simulink model "uasb_siso_simu"  (R2024b)
settings: Solver=VariableStepAuto  StartTime=0.0  StopTime=60  RelTol=1e-3
values from neighbouring files (symbols this model uses):
  A = blkdiag(A1, A2)    [generic_simo.m]    (also in uasb.m = [A1, zeros(3); uasb_identification.m = readmatrix('A2.csv'); uasb_siso.m = [-a_(2:end)', [1; 0]])
  B = [ ... (first row only)    [generic_simo.m]    (also in uasb.m = [B11(2:end), B12(2:end); uasb_identification.m = readmatrix('B2.csv'); uasb_siso.m = b')
  D = [D1 ... (first row only)    [generic_simo.m]    (also in uasb.m = [D1, zeros(3,1); uasb_siso.m = -a_(2:end)')
  delta = [1 -1]    [generic_simo.m]    (also in uasb.m = tf(1, delta, Ts, 'variable', 'z^-1'); uasb_siso.m = [1, -1])
  H = blkdiag(H1, H2)    [generic_simo.m]    (also in uasb.m = [H1, 0, 0, 0; uasb_siso.m = [1, 0])
  KE = K * E    [generic_simo.m]    (also in uasb.m = K*E; uasb_siso.m = K*E)
  KF = K * F    [generic_simo.m]    (also in uasb.m = K*F; uasb_siso.m = K*F)
  Kr = K * ones(ny*N, ny)    [generic_simo.m]    (also in uasb_siso.m = sum(K))
  Ts = 0.03    [generic_simo.m]    (also in uasb.m; uasb_identification.m = t(2) - t(1); uasb_siso.m = 1)
undefined symbols (not defined in the file or in its folder): a, a2, b, b2, dspblkCoreblockFVToolHelper, gcbh
settings Model: Creator=room2  LastModifiedBy=room2

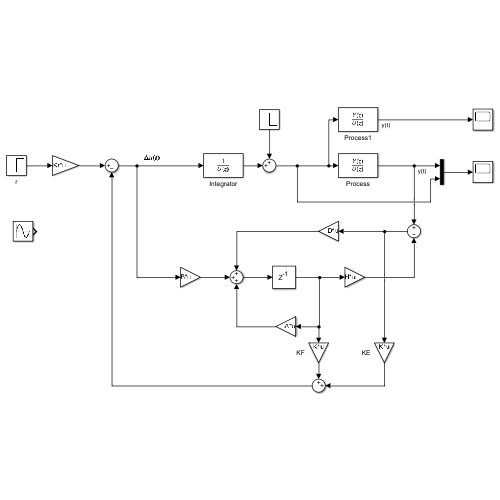
[thumbnail: Simulink's stored preview of the top-level diagram]
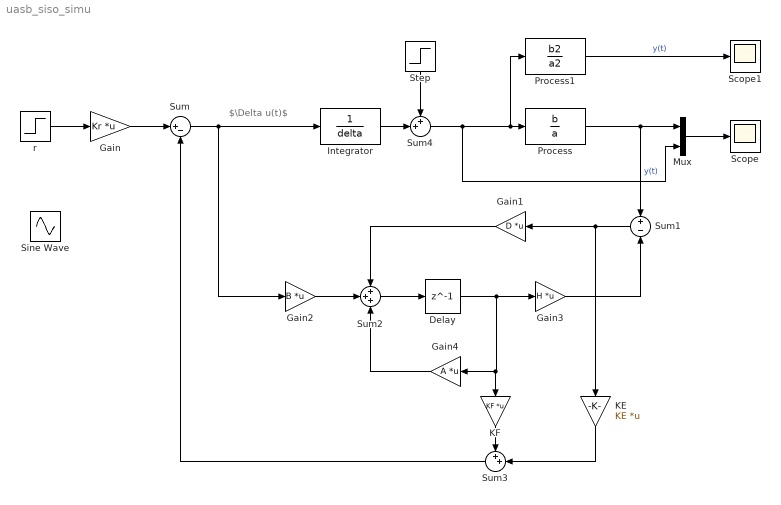
== system uasb_siso_simu ==
  note: $\Delta u(t)$
  Delay : Delay  DelayLength=1  SampleTime=Ts
  Gain : Gain  Gain=Kr  Multiplication=Matrix(K*u)
  Gain1 : Gain  Gain=D  Multiplication=Matrix(K*u)
  Gain2 : Gain  Gain=B  Multiplication=Matrix(K*u)
  Gain3 : Gain  Gain=H  Multiplication=Matrix(K*u)
  Gain4 : Gain  Gain=A  Multiplication=Matrix(K*u)
  Integrator : DiscreteTransferFcn  LoadFcn=dspblkCoreblockFVToolHelper(gcbh,'load');  Denominator=delta
      settings: CopyFcn=dspblkCoreblockFVToolHelper(gcbh,'copy');  DeleteFcn=dspblkCoreblockFVToolHelper(gcbh,'close');  ModelCloseFcn=dspblkCoreblockFVToolHelper(gcbh,'close');  PreSaveFcn=dspblkCoreblockFVToolHelper(gcbh,'presave');  PostSaveFcn=dspblkCoreblockFVToolHelper(gcbh,'postsave');  CloseFcn=dspblkCoreblockFVToolHelper(gcbh,'close');
  KE : Gain  Gain=KE  Multiplication=Matrix(K*u)
  KF : Gain  Gain=KF  Multiplication=Matrix(K*u)
  Mux : Mux  Inputs=2
  Process : DiscreteTransferFcn  LoadFcn=dspblkCoreblockFVToolHelper(gcbh,'load');  Numerator=b  Denominator=a
      settings: CopyFcn=dspblkCoreblockFVToolHelper(gcbh,'copy');  DeleteFcn=dspblkCoreblockFVToolHelper(gcbh,'close');  ModelCloseFcn=dspblkCoreblockFVToolHelper(gcbh,'close');  PreSaveFcn=dspblkCoreblockFVToolHelper(gcbh,'presave');  PostSaveFcn=dspblkCoreblockFVToolHelper(gcbh,'postsave');  CloseFcn=dspblkCoreblockFVToolHelper(gcbh,'close');
  Process1 : DiscreteTransferFcn  LoadFcn=dspblkCoreblockFVToolHelper(gcbh,'load');  Numerator=b2  Denominator=a2
      settings: CopyFcn=dspblkCoreblockFVToolHelper(gcbh,'copy');  DeleteFcn=dspblkCoreblockFVToolHelper(gcbh,'close');  ModelCloseFcn=dspblkCoreblockFVToolHelper(gcbh,'close');  PreSaveFcn=dspblkCoreblockFVToolHelper(gcbh,'presave');  PostSaveFcn=dspblkCoreblockFVToolHelper(gcbh,'postsave');  CloseFcn=dspblkCoreblockFVToolHelper(gcbh,'close');
  Scope : Scope
  Scope1 : Scope
  Sine Wave : Sin  Amplitude=1e-4  SampleTime=0
  Step : Step  Time=20  After=-0.1e-3  SampleTime=0
  Sum : Sum  Inputs=|+-
  Sum1 : Sum  Inputs=+|-
  Sum2 : Sum  Inputs=+++
  Sum3 : Sum  Inputs=++|
  Sum4 : Sum  Inputs=++|
  r : Step  Time=30  Before=1e-3  After=1.8e-3  SampleTime=0
  wires:
  r/1 -> Gain/1
  Gain/1 -> Sum/1
  Sum/1 -> Gain2/1, Integrator/1
  Sum1/1 -> Gain1/1, KE/1
  Gain1/1 -> Sum2/1
  Sum2/1 -> Delay/1
  Delay/1 -> KF/1, Gain4/1, Gain3/1
  Gain3/1 -> Sum1/2
  Gain4/1 -> Sum2/3
  KF/1 -> Sum3/1
  KE/1 -> Sum3/2
  Gain2/1 -> Sum2/2
  Sum3/1 -> Sum/2
  Process/1 -> Mux/1, Sum1/1  "y(t)"
  Mux/1 -> Scope/1
  Integrator/1 -> Sum4/2
  Sum4/1 -> Mux/2, Process1/1, Process/1
  Step/1 -> Sum4/1
  Process1/1 -> Scope1/1  "y(t)"
